simulink model "observateur_2020"  (Simulink 10.2)
settings: Solver=FixedStepAuto  StartTime=0.0  StopTime=inf  RelTol=1e-3  EnableMultiTasking=on
undefined symbols (not defined in the file): Aobs, Bobs, Cobs, Dobs, K_corr, S_corr, Te
libraries: legoev3lib x2
settings Model: Creator=carol  LastModifiedBy=carol  MultiThreadCoSim=auto  ExtModeTrigDuration=2
settings SolverCC: PositivePriorityOrder=on
settings DataIOCC: SaveFormat=Dataset  SignalLoggingSaveFormat=Dataset  ReturnWorkspaceOutputs=on
settings OptimizationCC: DefaultParameterBehavior=Inlined  EnhancedBackFolding=on  PassReuseOutputArgsAs=Individual arguments  ZeroExternalMemoryAtStartup=off  ZeroInternalMemoryAtStartup=off  LifeSpan=auto  MaxStackSize=64  OptimizeBlockOrder=speed  DifferentSizesBufferReuse=on  OptimizationCustomize=off  EfficientTunableParamExpr=on
settings DebuggingCC: UnderspecifiedInitializationDetection=Simplified  MergeDetectMultiDrivingBlocksExec=error  ParameterTunabilityLossMsg=error  FcnCallInpInsideContextMsg=error  UnconnectedInputMsg=none  UnconnectedOutputMsg=none  UnconnectedLineMsg=none  SFUnexpectedBacktrackingDiag=error  SFNoUnconditionalDefaultTransitionDiag=error  SFExecutionAtInitializationDiag=warning  ArithmeticOperatorsInVariantConditions=error
settings HardwareCC: ProdLargestAtomicInteger=Long  ProdLargestAtomicFloat=Float  ProdIntDivRoundTo=Zero  ProdEndianess=LittleEndian  ProdHWDeviceType=ARM Compatible->ARM 9  UseEmbeddedCoderFeatures=off  UseSimulinkCoderFeatures=off
settings ModelReferenceCC: EnableRefExpFcnMdlSchedulingChecks=off  PropagateSignalLabelsOutOfModel=on
settings SFSimCC: SimUseLocalCustomCode=on  MATLABDynamicMemAlloc=off  CustomCodeUndefinedFunction=FilterOut
settings RTWCC: Description=Embedded Coder  SystemTargetFile=ert.tlc  HardwareBoard=LEGO MINDSTORMS EV3  TLCOptions="-aInlineSetEventsForThisBaseRateFcn=TLC_FALSE -aSuppressMultiTaskScheduler=TLC_FALSE  -aRateBasedStepFcn=0"  TemplateMakefile=ert_default_tmf  RTWUseLocalCustomCode=on  Toolchain=Sourcery G++ Lite v2009q3  GPUComputeCapability=5.0
settings MATStruct: className=codertarget.tools.BuildHook  argsTopModelOnly=[]  excludedModels=[]  includeReferencedModels=on  includeTopModel=on  enabled=on  UseCoderTarget=[1]  TargetHardware=LEGO MINDSTORMS EV3  RTOS=Linux  RTOSBaseRateTaskPriority=40  DetectTaskOverruns=[0.0]  Scheduler_interrupt_source=[0.0]  DataVersion=2016.02  IPAddress=codertarget.ev3.internal.getEV3ExtmodeIPaddr  Port=17725  Verbose=[0]  Configuration=XCP on TCP/IP  signalBufferSize=[1000000.0]  BuildAction=Build, load and run  DisableParallelBuild=[0.0]  type=USB  deviceID=00aa00bb00cc  IPAddressCpy=192.168.1.2
settings CodeAppCC: ForceParamTrailComments=on  IgnoreCustomStorageClasses=off  OperatorAnnotations=on  SimulinkDataObjDesc=on  SFDataObjDesc=on  InsertBlockDesc=on  StateflowObjectComments=off
settings ERTTargetCC: SupportContinuousTime=on  SupportNonInlinedSFcns=on  SupportVariableSizeSignals=on  ExtModeTransport=2  ExtModeStaticAlloc=on  ExtModeMexFile=ext_xcp  ExtModeIntrfLevel=Level2 - Open  InlinedParameterPlacement=NonHierarchical
settings ConfigComp: CovMetricSettings=dwe  CovSaveCumulativeToWorkspaceVar=off  CovSaveSingleToWorkspaceVar=off  CovExternalEMLEnable=on  CovBoundaryAbsTol=1.0e-5
settings SettingsController: UseSoCProfilerForTargets=0

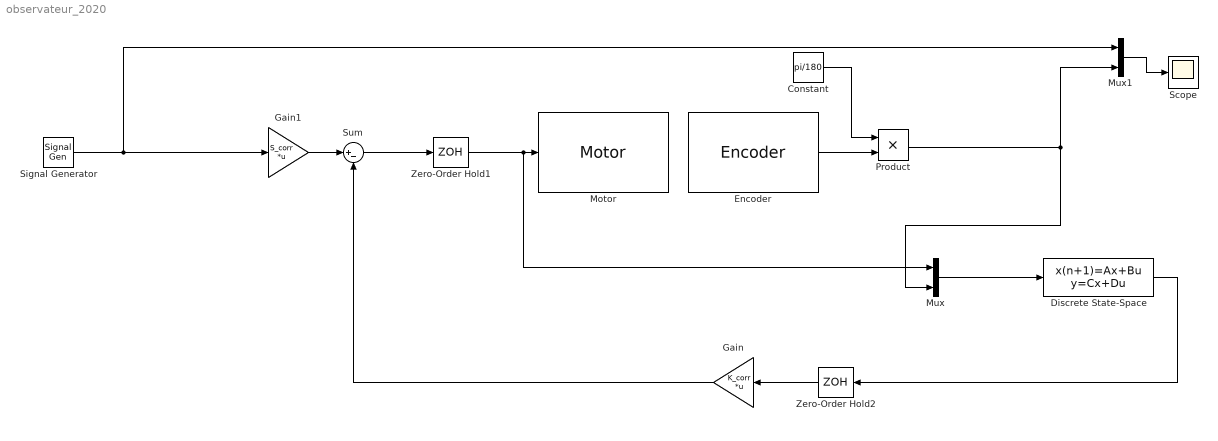
== system observateur_2020 ==
  Constant : Constant  Value=pi/180
  Discrete State-Space : DiscreteStateSpace  A=Aobs  B=Bobs  C=Cobs  D=Dobs  SampleTime=Te
  Encoder : legoev3lib/Encoder  portNumber=D  opMode=Reset by external signal  sampleTime=Te
  Gain : Gain  Gain=K_corr  Multiplication=Matrix(K*u)
  Gain1 : Gain  Gain=S_corr  Multiplication=Matrix(K*u)
  Motor : legoev3lib/Motor  sportNumber=D  sstopAction=Brake
  Mux : Mux  Inputs=2
  Mux1 : Mux  Inputs=2
  Product : Product
  Scope : Scope
  Signal Generator : SignalGenerator  WaveForm=square  Frequency=0.1
  Sum : Sum  Inputs=|+-
  Zero-Order Hold1 : ZeroOrderHold  SampleTime=Te
  Zero-Order Hold2 : ZeroOrderHold  SampleTime=Te
  wires:
  Encoder/1 -> Product/2
  Zero-Order Hold1/1 -> Mux/1, Motor/1
  Signal Generator/1 -> Mux1/1, Gain1/1
  Sum/1 -> Zero-Order Hold1/1
  Gain1/1 -> Sum/1
  Gain/1 -> Sum/2
  Product/1 -> Mux1/2, Mux/2
  Constant/1 -> Product/1
  Zero-Order Hold2/1 -> Gain/1
  Mux1/1 -> Scope/1
  Mux/1 -> Discrete State-Space/1
  Discrete State-Space/1 -> Zero-Order Hold2/1
